simulink model "gpucorr_txsim03r2"  (Simulink 7.4)
settings: Solver=ode3  SolverMode=SingleTasking  StartTime=0.0  StopTime=2^11  RelTol=1e-3
undefined symbols (not defined in the file): sfp
libraries: xbsIndex_r4 x296, xps_library x33, casper_library_misc x2
(part 1 of 2)
settings Model: Creator=gdesvignes  LastModifiedBy=jkocz

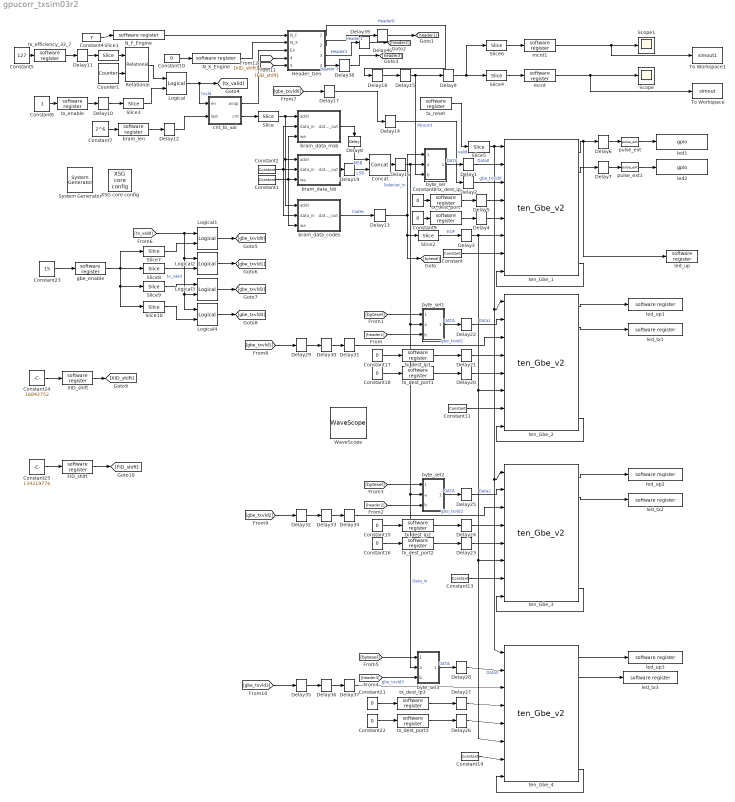
== system gpucorr_txsim03r2 ==
  " System Generator" : xbsIndex_r4/ System Generator  Tag=genX  SystemSampleTime=-1  xilinxfamily=virtex6  part=xc6vsx475t  speed=-1  package=ff1759  synthesis_tool=XST  clock_wrapper=Clock Enables  directory=./gpucorr_txsim03r2/sysgen  testbench=off  simulink_period=1  sysclk_period=5  dcm_input_clock_period=100  incr_netlist=off  trim_vbits=Everywhere in SubSystem  dbl_ovrd=According to Block Masks  core_generation=According to Block Masks  run_coregen=off  deprecated_control=off  eval_field=0  block_type=sysgen
      settings: block_version=11.4
  Concat : xbsIndex_r4/Concat  num_inputs=2  dbl_ovrd=off  block_type=concat
  Constant{,1,11,13,19} (5 alike) : xbsIndex_r4/Constant  arith_type=Boolean  const=0  n_bits=16  bin_pt=14  explicit_period=off  period=1  equ=P=C  opselect=C  inp2=PCIN>>17  opr=+  inp1=P  carry=CIN  dbl_ovrd=off  block_type=constant
      settings: block_version=11.4
  Constant{8..10,15..18,21..22} (9 alike) : Constant  Value=0
  Constant2 : xbsIndex_r4/Constant  arith_type=Unsigned  const=0  n_bits=32  bin_pt=0  explicit_period=off  period=1  equ=P=C  opselect=C  inp2=PCIN>>17  opr=+  inp1=P  carry=CIN  dbl_ovrd=off  block_type=constant
      settings: block_version=11.4
  Constant23 : Constant  Value=15
  Constant24 : Constant  Value=16842752
  Constant25 : Constant  Value=134219776
  Constant4 : Constant  Value=7
  Constant5 : Constant  Value=127
  Constant6 : Constant
  Constant7 : Constant  Value=2^6
  Counter1 : xbsIndex_r4/Counter  cnt_type=Free Running  cnt_to=Inf  operation=Up  start_count=0  cnt_by_val=1  arith_type=Unsigned  n_bits=7  bin_pt=0  load_pin=off  rst=off  en=off  explicit_period=on  period=1  dbl_ovrd=off  use_behavioral_HDL=off  implementation=Fabric  block_type=counter
      settings: block_version=11.4
  Delay{1..3,8,15,19,22,25,28,31,34,37..40} (15 alike) : xbsIndex_r4/Delay  en=off  latency=1  dbl_ovrd=off  reg_retiming=off  block_type=delay
      settings: block_version=11.4
  Delay{4..7,9..12,14,16..18,20..21,23..24,26..27,29..30,32..33,35..36} (24 alike) : xbsIndex_r4/Delay  en=off  latency=2  dbl_ovrd=off  reg_retiming=off  block_type=delay
      settings: block_version=11.4
  Delay13 : xbsIndex_r4/Delay  en=off  latency=3  dbl_ovrd=off  reg_retiming=off  block_type=delay
      settings: block_version=11.4
  FID_shift : xps_library/software register  Tag=xps:sw_reg  SystemSampleTime=-1  io_dir=From Processor  arith_type=Unsigned  bitwidth=32  bin_pt=0  sample_period=1  gw_name=gpucorr_txsim03r2_FID_shift_user_data_out
      link override gpucorr_txsim_tx_enable_user_data_out: arith_type=Unsigned  n_bits=32  bin_pt=0  period=1
  Header_Gen : Subsystem
  Logical{,1..4} (5 alike) : xbsIndex_r4/Logical  logical_function=AND  inputs=2  en=off  latency=0  precision=Full  arith_type=Unsigned  n_bits=16  bin_pt=0  align_bp=on  dbl_ovrd=off  block_type=logical
      settings: block_version=11.4
  N_F_Engine : xps_library/software register  Tag=xps:sw_reg  SystemSampleTime=-1  io_dir=From Processor  arith_type=Unsigned  bitwidth=32  bin_pt=0  sample_period=1  gw_name=gpucorr_txsim03r2_N_F_Engine_user_data_out
      link override gpucorr_txsim_N_F_Engine_user_data_out: arith_type=Unsigned  n_bits=32  bin_pt=0  period=1
  N_X_Engine : xps_library/software register  Tag=xps:sw_reg  SystemSampleTime=-1  io_dir=From Processor  arith_type=Unsigned  bitwidth=32  bin_pt=0  sample_period=1  gw_name=gpucorr_txsim03r2_N_X_Engine_user_data_out
      link override gpucorr_txsim_N_X_Engine_user_data_out: arith_type=Unsigned  n_bits=32  bin_pt=0  period=1
  Relational : xbsIndex_r4/Relational  mode=a>b  en=off  latency=1  dbl_ovrd=off  block_type=relational
  Scope : Scope
  Scope1 : Scope
      settings: TimeRange=100  YMin=-1  YMax=1
  Slice : xbsIndex_r4/Slice  nbits=15  boolean_output=off  mode=Lower Bit Location + Width  bit1=0  base1=MSB of Input  bit0=0  base0=LSB of Input  dbl_ovrd=off  block_type=slice
  Slice1 : xbsIndex_r4/Slice  nbits=7  boolean_output=off  mode=Lower Bit Location + Width  bit1=0  base1=MSB of Input  bit0=0  base0=LSB of Input  dbl_ovrd=off  block_type=slice
  Slice10 : xbsIndex_r4/Slice  nbits=15  boolean_output=on  mode=Lower Bit Location + Width  bit1=0  base1=MSB of Input  bit0=3  base0=LSB of Input  dbl_ovrd=off  block_type=slice
  Slice2 : xbsIndex_r4/Slice  nbits=15  boolean_output=on  mode=Upper Bit Location + Width  bit1=0  base1=MSB of Input  bit0=0  base0=LSB of Input  dbl_ovrd=off  block_type=slice
  Slice3 : xbsIndex_r4/Slice  nbits=15  boolean_output=on  mode=Lower Bit Location + Width  bit1=0  base1=MSB of Input  bit0=0  base0=LSB of Input  dbl_ovrd=off  block_type=slice
  Slice4 : xbsIndex_r4/Slice  nbits=32  boolean_output=off  mode=Lower Bit Location + Width  bit1=0  base1=MSB of Input  bit0=0  base0=LSB of Input  dbl_ovrd=off  block_type=slice
  Slice5 : xbsIndex_r4/Slice  nbits=15  boolean_output=on  mode=Lower Bit Location + Width  bit1=0  base1=MSB of Input  bit0=0  base0=LSB of Input  dbl_ovrd=off  block_type=slice
  Slice6 : xbsIndex_r4/Slice  nbits=32  boolean_output=off  mode=Upper Bit Location + Width  bit1=0  base1=MSB of Input  bit0=0  base0=MSB of Input  dbl_ovrd=off  block_type=slice
  Slice7 : xbsIndex_r4/Slice  nbits=15  boolean_output=on  mode=Lower Bit Location + Width  bit1=0  base1=MSB of Input  bit0=0  base0=LSB of Input  dbl_ovrd=off  block_type=slice
  Slice8 : xbsIndex_r4/Slice  nbits=15  boolean_output=on  mode=Lower Bit Location + Width  bit1=0  base1=MSB of Input  bit0=1  base0=LSB of Input  dbl_ovrd=off  block_type=slice
  Slice9 : xbsIndex_r4/Slice  nbits=15  boolean_output=on  mode=Lower Bit Location + Width  bit1=0  base1=MSB of Input  bit0=2  base0=LSB of Input  dbl_ovrd=off  block_type=slice
  To Workspace : ToWorkspace  VariableName=simout  SampleTime=-1  SaveFormat=Structure
  To Workspace1 : ToWorkspace  VariableName=simout1  SampleTime=-1  SaveFormat=Structure
  WaveScope : xbsIndex_r4/WaveScope  block_type=wavescope
      settings: block_version=11.4
  XID_shift : xps_library/software register  Tag=xps:sw_reg  SystemSampleTime=-1  io_dir=From Processor  arith_type=Unsigned  bitwidth=32  bin_pt=0  sample_period=1  gw_name=gpucorr_txsim03r2_XID_shift_user_data_out
      link override gpucorr_txsim_tx_enable_user_data_out: arith_type=Unsigned  n_bits=32  bin_pt=0  period=1
  XSG core config : xps_library/XSG core config  Tag=xps:xsg  SystemSampleTime=-1  hw_sys=ROACH2:sx475t  clk_src=sys_clk  ROACH_clk_src=sys_clk2x  ROACH2_clk_src=sys_clk  clk_rate=200  sample_period=1  synthesis_tool=XST
  bram_data_codes : Subsystem  Tag=xps:bram  AncestorBlock=xps_library/Shared BRAM  mask{arith_type=Unsigned, addr_width=12, data_width=32, data_bin_pt=0, init_vals=[255,2147483648], sample_rate=1}
      mask prompts: arith_type "Output Data Type"; addr_width "Address width"; data_width "Data Width"; data_bin_pt "Data Binary Point"; init_vals "Initial 32-bit values (simulation only)"; sample_rate "Sample rate"
      mask init:
      | shared_bram_mask;
      mask StyleString: popup(Unsigned|Signed  (2's comp)),edit,popup(8|16|32|64|128),edit,edit,edit
  bram_data_lsb : Subsystem  Tag=xps:bram  AncestorBlock=xps_library/Shared BRAM  mask{arith_type=Unsigned, addr_width=12, data_width=32, data_bin_pt=0, init_vals=[216,212,216], sample_rate=1}
      mask prompts: arith_type "Output Data Type"; addr_width "Address width"; data_width "Data Width"; data_bin_pt "Data Binary Point"; init_vals "Initial 32-bit values (simulation only)"; sample_rate "Sample rate"
      mask init:
      | shared_bram_mask;
      mask StyleString: popup(Unsigned|Signed  (2's comp)),edit,popup(8|16|32|64|128),edit,edit,edit
  bram_data_msb : Subsystem  Tag=xps:bram  AncestorBlock=xps_library/Shared BRAM  mask{arith_type=Unsigned, addr_width=12, data_width=32, data_bin_pt=0, init_vals=[116,112,116], sample_rate=1}
      mask prompts: arith_type "Output Data Type"; addr_width "Address width"; data_width "Data Width"; data_bin_pt "Data Binary Point"; init_vals "Initial 32-bit values (simulation only)"; sample_rate "Sample rate"
      mask init:
      | shared_bram_mask;
      mask StyleString: popup(Unsigned|Signed  (2's comp)),edit,popup(8|16|32|64|128),edit,edit,edit
  bram_len : xps_library/software register  Tag=xps:sw_reg  SystemSampleTime=-1  io_dir=From Processor  arith_type=Unsigned  bitwidth=32  bin_pt=0  sample_period=1  gw_name=gpucorr_txsim03r2_bram_len_user_data_out
      link override gpucorr_txsim_bram_len_user_data_out: arith_type=Unsigned  n_bits=32  bin_pt=0  period=1
  byte_sel : Subsystem
  byte_sel1 : Subsystem
  byte_sel2 : Subsystem
  byte_sel3 : Subsystem
  cnt_to_val : Subsystem
  gbe_enable : xps_library/software register  Tag=xps:sw_reg  SystemSampleTime=-1  io_dir=From Processor  arith_type=Unsigned  bitwidth=32  bin_pt=0  sample_period=1  gw_name=gpucorr_txsim03r2_gbe_enable_user_data_out
      link override gpucorr_txsim_tx_enable_user_data_out: arith_type=Unsigned  n_bits=32  bin_pt=0  period=1
  led1 : xps_library/gpio  Tag=xps:gpio  SystemSampleTime=-1  io_group=ROACH:led  io_dir=out  arith_type=Boolean  bitwidth=1  bin_pt=0  bit_index=1  sample_period=1  use_single_ended=off  use_ddr=off  reg_iob=on  reg_clk_phase=0  termination=None
      link override convert: arith_type=Boolean  n_bits=1  bin_pt=0
  led2 : xps_library/gpio  Tag=xps:gpio  SystemSampleTime=-1  io_group=ROACH:led  io_dir=out  arith_type=Boolean  bitwidth=1  bin_pt=0  bit_index=2  sample_period=1  use_single_ended=off  use_ddr=off  reg_iob=on  reg_clk_phase=0  termination=None
      link override convert: arith_type=Boolean  n_bits=1  bin_pt=0
  led_tx1 : xps_library/software register  Tag=xps:sw_reg  SystemSampleTime=-1  io_dir=To Processor  arith_type=Unsigned  bitwidth=32  bin_pt=0  sample_period=1  gw_name=gpucorr_txsim03r2_led_tx1_user_data_in
      link override convert: arith_type=Unsigned  n_bits=32  bin_pt=0
  led_tx2 : xps_library/software register  Tag=xps:sw_reg  SystemSampleTime=-1  io_dir=To Processor  arith_type=Unsigned  bitwidth=32  bin_pt=0  sample_period=1  gw_name=gpucorr_txsim03r2_led_tx2_user_data_in
      link override convert: arith_type=Unsigned  n_bits=32  bin_pt=0
  led_tx3 : xps_library/software register  Tag=xps:sw_reg  SystemSampleTime=-1  io_dir=To Processor  arith_type=Unsigned  bitwidth=32  bin_pt=0  sample_period=1  gw_name=gpucorr_txsim03r2_led_tx3_user_data_in
      link override convert: arith_type=Unsigned  n_bits=32  bin_pt=0
  led_up : xps_library/software register  Tag=xps:sw_reg  SystemSampleTime=-1  io_dir=To Processor  arith_type=Unsigned  bitwidth=32  bin_pt=0  sample_period=1  gw_name=gpucorr_txsim03r2_led_up_user_data_in
      link override convert: arith_type=Unsigned  n_bits=32  bin_pt=0
  led_up1 : xps_library/software register  Tag=xps:sw_reg  SystemSampleTime=-1  io_dir=To Processor  arith_type=Unsigned  bitwidth=32  bin_pt=0  sample_period=1  gw_name=gpucorr_txsim03r2_led_up1_user_data_in
      link override convert: arith_type=Unsigned  n_bits=32  bin_pt=0
  led_up2 : xps_library/software register  Tag=xps:sw_reg  SystemSampleTime=-1  io_dir=To Processor  arith_type=Unsigned  bitwidth=32  bin_pt=0  sample_period=1  gw_name=gpucorr_txsim03r2_led_up2_user_data_in
      link override convert: arith_type=Unsigned  n_bits=32  bin_pt=0
  led_up3 : xps_library/software register  Tag=xps:sw_reg  SystemSampleTime=-1  io_dir=To Processor  arith_type=Unsigned  bitwidth=32  bin_pt=0  sample_period=1  gw_name=gpucorr_txsim03r2_led_up3_user_data_in
      link override convert: arith_type=Unsigned  n_bits=32  bin_pt=0
  mcnt : xps_library/software register  Tag=xps:sw_reg  SystemSampleTime=-1  io_dir=To Processor  arith_type=Unsigned  bitwidth=32  bin_pt=0  sample_period=1  gw_name=gpucorr_txsim03r2_mcnt_user_data_in
      link override convert: arith_type=Unsigned  n_bits=32  bin_pt=0
  mcnt1 : xps_library/software register  Tag=xps:sw_reg  SystemSampleTime=-1  io_dir=To Processor  arith_type=Unsigned  bitwidth=32  bin_pt=0  sample_period=1  gw_name=gpucorr_txsim03r2_mcnt1_user_data_in
      link override convert: arith_type=Unsigned  n_bits=32  bin_pt=0
  pulse_ext : casper_library_misc/pulse_ext  SystemSampleTime=-1  pulse_len=5
  pulse_ext1 : casper_library_misc/pulse_ext  SystemSampleTime=-1  pulse_len=5
  ten_Gbe_1 : xps_library/ten_Gbe_v2  Tag=xps:tengbe_v2  SystemSampleTime=-1  flavour=sfp+  slot=0  port_r1=0  port_r2_cx4=0  port_r2_sfpp=0  rx_dist_ram=on  large_frames=on  show_param=on  pre_emph_r2=0.74  pre_emph=3  post_emph_r2=0.18  rxeqmix_r2=7  swing_r2=940  swing=800  fab_en=on  fab_mac=hex2dec('123456780000')  fab_ip=192*(2^24) + 168*(2^16) + 5*(2^8) + 20*(2^0)  fab_udp=10000  fab_gate=1  cpu_rx_en=on  cpu_tx_en=on
  ten_Gbe_2 : xps_library/ten_Gbe_v2  Tag=xps:tengbe_v2  SystemSampleTime=-1  flavour=sfp+  slot=0  port_r1=0  port_r2_cx4=0  port_r2_sfpp=1  rx_dist_ram=on  large_frames=on  show_param=on  pre_emph_r2=0.74  pre_emph=3  post_emph_r2=0.18  rxeqmix_r2=7  swing_r2=940  swing=800  fab_en=on  fab_mac=hex2dec('123456789000')  fab_ip=192*(2^24) + 168*(2^16) + 5*(2^8) + 21*(2^0)  fab_udp=10001  fab_gate=1  cpu_rx_en=on  cpu_tx_en=on
  ten_Gbe_3 : xps_library/ten_Gbe_v2  Tag=xps:tengbe_v2  SystemSampleTime=-1  flavour=sfp+  slot=0  port_r1=0  port_r2_cx4=0  port_r2_sfpp=2  rx_dist_ram=on  large_frames=on  show_param=on  pre_emph_r2=0.74  pre_emph=3  post_emph_r2=0.18  rxeqmix_r2=7  swing_r2=940  swing=800  fab_en=on  fab_mac=hex2dec('123456780900')  fab_ip=192*(2^24) + 168*(2^16) + 5*(2^8) + 22*(2^0)  fab_udp=10002  fab_gate=1  cpu_rx_en=on  cpu_tx_en=on
  ten_Gbe_4 : xps_library/ten_Gbe_v2  Tag=xps:tengbe_v2  SystemSampleTime=-1  flavour=sfp+  slot=0  port_r1=0  port_r2_cx4=0  port_r2_sfpp=3  rx_dist_ram=on  large_frames=on  show_param=on  pre_emph_r2=0.74  pre_emph=3  post_emph_r2=0.18  rxeqmix_r2=7  swing_r2=940  swing=800  fab_en=on  fab_mac=hex2dec('123456780090')  fab_ip=192*(2^24) + 168*(2^16) + 5*(2^8) + 23*(2^0)  fab_udp=10003  fab_gate=1  cpu_rx_en=on  cpu_tx_en=on
  tx_dest_ip : xps_library/software register  Tag=xps:sw_reg  SystemSampleTime=-1  io_dir=From Processor  arith_type=Unsigned  bitwidth=32  bin_pt=0  sample_period=1  gw_name=gpucorr_txsim03r2_tx_dest_ip_user_data_out
      link override gpucorr_txsim_tx_dest_ip_user_data_out: arith_type=Unsigned  n_bits=32  bin_pt=0  period=1
  tx_dest_ip1 : xps_library/software register  Tag=xps:sw_reg  SystemSampleTime=-1  io_dir=From Processor  arith_type=Unsigned  bitwidth=32  bin_pt=0  sample_period=1  gw_name=gpucorr_txsim03r2_tx_dest_ip1_user_data_out
      link override gpucorr_txsim_tx_dest_ip_user_data_out: arith_type=Unsigned  n_bits=32  bin_pt=0  period=1
  tx_dest_ip2 : xps_library/software register  Tag=xps:sw_reg  SystemSampleTime=-1  io_dir=From Processor  arith_type=Unsigned  bitwidth=32  bin_pt=0  sample_period=1  gw_name=gpucorr_txsim03r2_tx_dest_ip2_user_data_out
      link override gpucorr_txsim_tx_dest_ip_user_data_out: arith_type=Unsigned  n_bits=32  bin_pt=0  period=1
  tx_dest_ip3 : xps_library/software register  Tag=xps:sw_reg  SystemSampleTime=-1  io_dir=From Processor  arith_type=Unsigned  bitwidth=32  bin_pt=0  sample_period=1  gw_name=gpucorr_txsim03r2_tx_dest_ip3_user_data_out
      link override gpucorr_txsim_tx_dest_ip_user_data_out: arith_type=Unsigned  n_bits=32  bin_pt=0  period=1
  tx_dest_port : xps_library/software register  Tag=xps:sw_reg  SystemSampleTime=-1  io_dir=From Processor  arith_type=Unsigned  bitwidth=32  bin_pt=0  sample_period=1  gw_name=gpucorr_txsim03r2_tx_dest_port_user_data_out
      link override gpucorr_txsim_tx_dest_port_user_data_out: arith_type=Unsigned  n_bits=32  bin_pt=0  period=1
  tx_dest_port1 : xps_library/software register  Tag=xps:sw_reg  SystemSampleTime=-1  io_dir=From Processor  arith_type=Unsigned  bitwidth=32  bin_pt=0  sample_period=1  gw_name=gpucorr_txsim03r2_tx_dest_port1_user_data_out
      link override gpucorr_txsim_tx_dest_port_user_data_out: arith_type=Unsigned  n_bits=32  bin_pt=0  period=1
  tx_dest_port2 : xps_library/software register  Tag=xps:sw_reg  SystemSampleTime=-1  io_dir=From Processor  arith_type=Unsigned  bitwidth=32  bin_pt=0  sample_period=1  gw_name=gpucorr_txsim03r2_tx_dest_port2_user_data_out
      link override gpucorr_txsim_tx_dest_port_user_data_out: arith_type=Unsigned  n_bits=32  bin_pt=0  period=1
  tx_dest_port3 : xps_library/software register  Tag=xps:sw_reg  SystemSampleTime=-1  io_dir=From Processor  arith_type=Unsigned  bitwidth=32  bin_pt=0  sample_period=1  gw_name=gpucorr_txsim03r2_tx_dest_port3_user_data_out
      link override gpucorr_txsim_tx_dest_port_user_data_out: arith_type=Unsigned  n_bits=32  bin_pt=0  period=1
  tx_efficiency_32_7 : xps_library/software register  Tag=xps:sw_reg  SystemSampleTime=-1  io_dir=From Processor  arith_type=Unsigned  bitwidth=32  bin_pt=0  sample_period=1  gw_name=gpucorr_txsim03r2_tx_efficiency_32_7_user_data_out
      link override gpucorr_txsim_tx_efficiency_32_7_user_data_out: arith_type=Unsigned  n_bits=32  bin_pt=0  period=1
  tx_enable : xps_library/software register  Tag=xps:sw_reg  SystemSampleTime=-1  io_dir=From Processor  arith_type=Unsigned  bitwidth=32  bin_pt=0  sample_period=1  gw_name=gpucorr_txsim03r2_tx_enable_user_data_out
      link override gpucorr_txsim_tx_enable_user_data_out: arith_type=Unsigned  n_bits=32  bin_pt=0  period=1
  tx_reset : xps_library/software register  Tag=xps:sw_reg  SystemSampleTime=-1  io_dir=From Processor  arith_type=Unsigned  bitwidth=32  bin_pt=0  sample_period=1  gw_name=gpucorr_txsim03r2_tx_reset_user_data_out
      link override gpucorr_txsim_tx_reset_user_data_out: arith_type=Unsigned  n_bits=32  bin_pt=0  period=1
  wires:
  tx_dest_ip/1 -> Delay5/1
  tx_dest_port/1 -> Delay4/1
  Slice/1 -> bram_data_lsb/1(addr), bram_data_codes/1(addr), bram_data_msb/1(addr)
  Constant1/1 -> bram_data_lsb/3(we), bram_data_msb/3(we), bram_data_codes/3(we)
  Constant2/1 -> bram_data_lsb/2(data_in), bram_data_msb/2(data_in), bram_data_codes/2(data_in)
  bram_data_msb/1(data_out) -> Delay8/1
  tx_efficiency_32_7/1 -> Delay11/1
  Slice1/1 -> Relational/1
  Counter1/1 -> Relational/2
  bram_len/1 -> Delay12/1
  cnt_to_val/1(wrap) -> Header_Gen/3(En)
  Concat/1 -> Delay16/1
  bram_data_codes/1(data_out) -> Delay13/1  "Codes"
  byte_sel/1(dout) -> Delay1/1  "DATA"
  Delay17/1 -> Delay14/1
  Slice2/1 -> Delay3/1  "EOF"
  tx_enable/1 -> Delay10/1
  Logical/1 -> cnt_to_val/1(en), [tx_valid]  "txvld"
  Relational/1 -> Logical/1
  Slice3/1 -> Logical/2
  Constant5/1 -> tx_efficiency_32_7/1
  Constant6/1 -> tx_enable/1
  Constant7/1 -> bram_len/1
  Constant8/1 -> tx_dest_ip/1
  Constant9/1 -> tx_dest_port/1
  Slice4/1 -> mcnt/1
  Delay6/1 -> pulse_ext/1
  Delay7/1 -> pulse_ext1/1
  Delay9/1 -> Slice4/1, Slice6/1
  Delay10/1 -> Slice3/1
  Delay11/1 -> Slice1/1
  Delay12/1 -> cnt_to_val/2(last)
  Delay13/1 -> byte_sel/1(byte_sel), Slice2/1, [bytesel]  "Selecter_in"
  Delay14/1 -> Delay2/1  "valid"
  Delay15/1 -> byte_sel/3(b), Delay9/1  "Mcount"
  Delay16/1 -> byte_sel1/2(a), byte_sel2/2(a), byte_sel3/2(a), byte_sel/2(a)  "Data_in"
  Delay18/1 -> Delay15/1
  tx_reset/1 -> Slice5/1
  Slice5/1 -> ten_Gbe_4/1, ten_Gbe_3/1, ten_Gbe_2/1, ten_Gbe_1/1
  Constant/1 -> ten_Gbe_1/7
  Delay1/1 -> ten_Gbe_1/2  "Data0"
  Delay2/1 -> ten_Gbe_1/3  "gbe_txvld0"
  ten_Gbe_1/1 -> Delay6/1, led_up/1
  pulse_ext/1 -> led1/1
  pulse_ext1/1 -> led2/1
  Delay5/1 -> ten_Gbe_1/4
  Delay4/1 -> ten_Gbe_1/5
  Delay3/1 -> ten_Gbe_4/6, ten_Gbe_3/6, ten_Gbe_2/6, ten_Gbe_1/6
  ten_Gbe_1/3 -> Delay7/1
  cnt_to_val/2(cnt) -> Slice/1
  Constant4/1 -> N_F_Engine/1
  Constant10/1 -> N_X_Engine/1
  N_X_Engine/1 -> Header_Gen/2(N_X)
  Header_Gen/1(Header) -> Delay18/1  "Header0"
  mcnt/1 -> Scope/1, To Workspace/1
  Slice6/1 -> mcnt1/1
  mcnt1/1 -> Scope1/1, To Workspace1/1
  Delay8/1 -> Concat/1  "MSB"
  bram_data_lsb/1(data_out) -> Delay19/1
  Delay19/1 -> Concat/2  "LSB"
  Constant11/1 -> ten_Gbe_2/7
  tx_dest_ip1/1 -> Delay21/1
  tx_dest_port1/1 -> Delay20/1
  Constant17/1 -> tx_dest_ip1/1
  Constant18/1 -> tx_dest_port1/1
  Delay21/1 -> ten_Gbe_2/4
  Delay20/1 -> ten_Gbe_2/5
  ten_Gbe_2/1 -> led_up1/1
  ten_Gbe_2/3 -> led_tx1/1
  byte_sel1/1(dout) -> Delay22/1  "DATA"
  Delay22/1 -> ten_Gbe_2/2  "Data1"
  [bytesel] -> byte_sel1/1(byte_sel)
  [header1] -> byte_sel1/3(b)
  N_F_Engine/1 -> Header_Gen/1(N_F)
  Constant13/1 -> ten_Gbe_3/7
  tx_dest_ip2/1 -> Delay24/1
  tx_dest_port2/1 -> Delay23/1
  Constant15/1 -> tx_dest_ip2/1
  Constant16/1 -> tx_dest_port2/1
  Delay24/1 -> ten_Gbe_3/4
  Delay23/1 -> ten_Gbe_3/5
  ten_Gbe_3/1 -> led_up2/1
  ten_Gbe_3/3 -> led_tx2/1
  byte_sel2/1(dout) -> Delay25/1  "DATA"
  Delay25/1 -> ten_Gbe_3/2  "Data2"
  [bytesel] -> byte_sel2/1(byte_sel)
  [header2] -> byte_sel2/3(b)
  Constant19/1 -> ten_Gbe_4/7
  tx_dest_ip3/1 -> Delay27/1
  tx_dest_port3/1 -> Delay26/1
  Constant21/1 -> tx_dest_ip3/1
  Constant22/1 -> tx_dest_port3/1
  Delay27/1 -> ten_Gbe_4/4
  Delay26/1 -> ten_Gbe_4/5
  ten_Gbe_4/1 -> led_up3/1
  byte_sel3/1(dout) -> Delay28/1  "DATA"
  Delay28/1 -> ten_Gbe_4/2  "Data3"
  [bytesel] -> byte_sel3/1(byte_sel)
  [header3] -> byte_sel3/3(b)
  Constant23/1 -> gbe_enable/1
  gbe_enable/1 -> Slice7/1, Slice8/1, Slice9/1, Slice10/1
  Slice7/1 -> Logical1/2
  Slice8/1 -> Logical2/2
  Slice9/1 -> Logical3/1
  Slice10/1 -> Logical4/2
  [tx_valid] -> Logical1/1, Logical2/1, Logical3/2, Logical4/1  "tx_valid"
  Logical1/1 -> [gbe_txvld0]
  Logical2/1 -> [gbe_txvld1]
  Logical3/1 -> [gbe_txvld2]
  Logical4/1 -> [gbe_txvld3]
  [gbe_txvld0] -> Delay17/1
  [gbe_txvld1] -> Delay29/1
  Delay29/1 -> Delay30/1
  Delay30/1 -> Delay31/1
  [gbe_txvld2] -> Delay32/1
  Delay32/1 -> Delay33/1
  Delay33/1 -> Delay34/1
  [gbe_txvld3] -> Delay35/1
  Delay35/1 -> Delay36/1
  Delay36/1 -> Delay37/1
  Delay31/1 -> ten_Gbe_2/3  "gbe_txvld1"
  Delay34/1 -> ten_Gbe_3/3  "gbe_txvld2"
  Delay37/1 -> ten_Gbe_4/3  "gbe_txvld3"
  Delay38/1 -> [header3]
  Header_Gen/4(Header3) -> Delay38/1  "Header 3"
  Delay40/1 -> [header1]
  Header_Gen/2(Header1) -> Delay40/1  "Header1"
  Header_Gen/3(Header2) -> Delay39/1  "Header2"
  Delay39/1 -> [header2]
  [FID_shift] -> Header_Gen/4(FID_shift)
  [XID_shift] -> Header_Gen/5(XID_shift)
  XID_shift/1 -> [XID_shift]
  FID_shift/1 -> [FID_shift]
  Constant24/1 -> XID_shift/1
  Constant25/1 -> FID_shift/1
  ten_Gbe_4/3 -> led_tx3/1
  ten_Gbe_4/12 -> ten_Gbe_4/8
  ten_Gbe_3/12 -> ten_Gbe_3/8
  ten_Gbe_2/12 -> ten_Gbe_2/8
  ten_Gbe_1/12 -> ten_Gbe_1/8

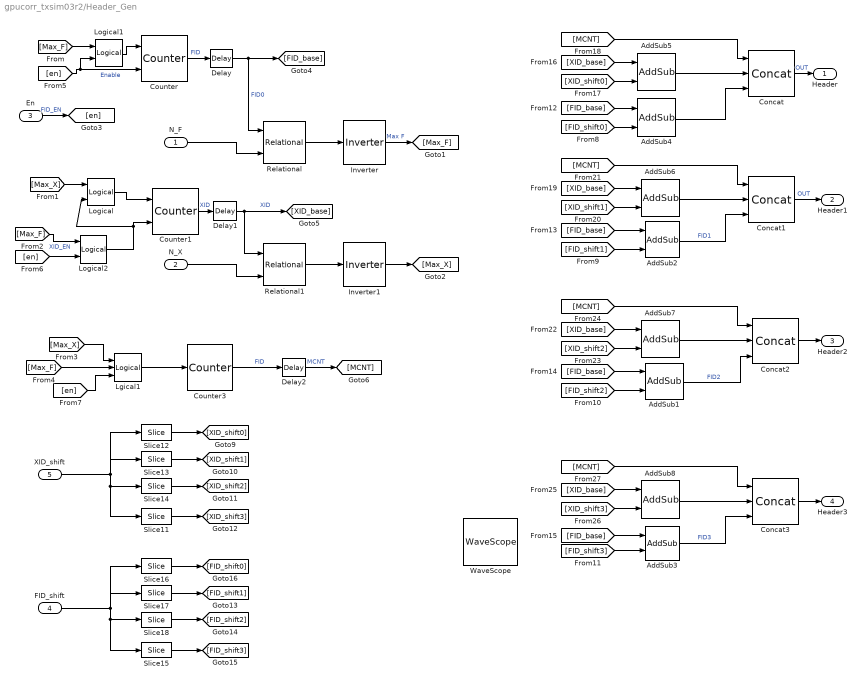
== system gpucorr_txsim03r2/Header_Gen ==
  N_F : Inport
  N_X : Inport  Port=2
  En : Inport  Port=3
  FID_shift : Inport  Port=4
  XID_shift : Inport  Port=5
  AddSub{1..8} (8 alike) : xbsIndex_r4/AddSub  mode=Addition  use_carryin=off  use_carryout=off  en=off  latency=0  precision=User Defined  arith_type=Unsigned  n_bits=8  bin_pt=0  quantization=Truncate  overflow=Wrap  dbl_ovrd=off  use_behavioral_HDL=off  hw_selection=Fabric  pipelined=off  block_type=addsub
  Concat{,1..3} (4 alike) : xbsIndex_r4/Concat  num_inputs=3  dbl_ovrd=off  block_type=concat
  Counter : xbsIndex_r4/Counter  cnt_type=Free Running  cnt_to=Inf  operation=Up  start_count=0  cnt_by_val=1  arith_type=Unsigned  n_bits=8  bin_pt=0  load_pin=off  rst=on  en=on  explicit_period=on  period=1  dbl_ovrd=off  use_behavioral_HDL=off  implementation=Fabric  block_type=counter
      settings: block_version=11.4
  Counter1 : xbsIndex_r4/Counter  cnt_type=Free Running  cnt_to=Inf  operation=Up  start_count=0  cnt_by_val=1  arith_type=Unsigned  n_bits=8  bin_pt=0  load_pin=off  rst=on  en=on  explicit_period=on  period=1  dbl_ovrd=off  use_behavioral_HDL=off  implementation=Fabric  block_type=counter
      settings: block_version=11.4
  Counter3 : xbsIndex_r4/Counter  cnt_type=Free Running  cnt_to=Inf  operation=Up  start_count=0  cnt_by_val=1  arith_type=Unsigned  n_bits=48  bin_pt=0  load_pin=off  rst=off  en=on  explicit_period=on  period=1  dbl_ovrd=off  use_behavioral_HDL=off  implementation=Fabric  block_type=counter
      settings: block_version=11.4
  Delay : xbsIndex_r4/Delay  en=off  latency=1  dbl_ovrd=off  reg_retiming=off  block_type=delay
      settings: block_version=11.4
  Delay1 : xbsIndex_r4/Delay  en=off  latency=1  dbl_ovrd=off  reg_retiming=off  block_type=delay
      settings: block_version=11.4
  Delay2 : xbsIndex_r4/Delay  en=off  latency=1  dbl_ovrd=off  reg_retiming=off  block_type=delay
      settings: block_version=11.4
  Inverter : xbsIndex_r4/Inverter  en=off  latency=0  dbl_ovrd=off  block_type=inv
      settings: block_version=11.4
  Inverter1 : xbsIndex_r4/Inverter  en=off  latency=0  dbl_ovrd=off  block_type=inv
      settings: block_version=11.4
  Lgical1 : xbsIndex_r4/Logical  logical_function=AND  inputs=3  en=off  latency=0  precision=Full  arith_type=Unsigned  n_bits=16  bin_pt=0  align_bp=on  dbl_ovrd=off  block_type=logical
      settings: block_version=11.4
  Logical : xbsIndex_r4/Logical  logical_function=AND  inputs=2  en=off  latency=0  precision=Full  arith_type=Unsigned  n_bits=16  bin_pt=0  align_bp=on  dbl_ovrd=off  block_type=logical
      settings: block_version=11.4
  Logical1 : xbsIndex_r4/Logical  logical_function=AND  inputs=2  en=off  latency=0  precision=Full  arith_type=Unsigned  n_bits=16  bin_pt=0  align_bp=on  dbl_ovrd=off  block_type=logical
      settings: block_version=11.4
  Logical2 : xbsIndex_r4/Logical  logical_function=AND  inputs=2  en=off  latency=0  precision=Full  arith_type=Unsigned  n_bits=16  bin_pt=0  align_bp=on  dbl_ovrd=off  block_type=logical
      settings: block_version=11.4
  Relational : xbsIndex_r4/Relational  mode=a<b  en=off  latency=0  dbl_ovrd=off  block_type=relational
  Relational1 : xbsIndex_r4/Relational  mode=a<b  en=off  latency=0  dbl_ovrd=off  block_type=relational
  Slice11 : xbsIndex_r4/Slice  nbits=8  boolean_output=off  mode=Lower Bit Location + Width  bit1=0  base1=MSB of Input  bit0=24  base0=LSB of Input  dbl_ovrd=off  block_type=slice
  Slice12 : xbsIndex_r4/Slice  nbits=8  boolean_output=off  mode=Lower Bit Location + Width  bit1=0  base1=MSB of Input  bit0=0  base0=LSB of Input  dbl_ovrd=off  block_type=slice
  Slice13 : xbsIndex_r4/Slice  nbits=8  boolean_output=off  mode=Lower Bit Location + Width  bit1=0  base1=MSB of Input  bit0=8  base0=LSB of Input  dbl_ovrd=off  block_type=slice
  Slice14 : xbsIndex_r4/Slice  nbits=8  boolean_output=off  mode=Lower Bit Location + Width  bit1=0  base1=MSB of Input  bit0=16  base0=LSB of Input  dbl_ovrd=off  block_type=slice
  Slice15 : xbsIndex_r4/Slice  nbits=8  boolean_output=off  mode=Lower Bit Location + Width  bit1=0  base1=MSB of Input  bit0=24  base0=LSB of Input  dbl_ovrd=off  block_type=slice
  Slice16 : xbsIndex_r4/Slice  nbits=8  boolean_output=off  mode=Lower Bit Location + Width  bit1=0  base1=MSB of Input  bit0=0  base0=LSB of Input  dbl_ovrd=off  block_type=slice
  Slice17 : xbsIndex_r4/Slice  nbits=8  boolean_output=off  mode=Lower Bit Location + Width  bit1=0  base1=MSB of Input  bit0=8  base0=LSB of Input  dbl_ovrd=off  block_type=slice
  Slice18 : xbsIndex_r4/Slice  nbits=8  boolean_output=off  mode=Lower Bit Location + Width  bit1=0  base1=MSB of Input  bit0=16  base0=LSB of Input  dbl_ovrd=off  block_type=slice
  WaveScope : xbsIndex_r4/WaveScope  block_type=wavescope
      settings: block_version=11.4
  Header : Outport
  Header1 : Outport  Port=2
  Header2 : Outport  Port=3
  Header3 : Outport  Port=4
  wires:
  Counter/1 -> Delay/1  "FID"
  Relational/1 -> Inverter/1
  Counter1/1 -> Delay1/1  "XID"
  Relational1/1 -> Inverter1/1
  N_F/1 -> Relational/2
  Inverter/1 -> [Max_F]  "Max F"
  Inverter1/1 -> [Max_X]
  [Max_F] -> Logical2/1  "XID_EN"
  [Max_X] -> Logical/1
  Logical/1 -> Counter1/1
  [Max_X] -> Lgical1/1
  Concat/1 -> Header/1  "OUT"
  N_X/1 -> Relational1/2
  Counter3/1 -> Delay2/1  "FID"
  En/1 -> [en]  "FID_EN"
  [Max_F] -> Logical1/1
  [en] -> Logical1/2, Counter/2  "Enable"
  Logical1/1 -> Counter/1
  [en] -> Logical2/2
  Logical2/1 -> Counter1/2, Logical/2
  [Max_F] -> Lgical1/2
  [en] -> Lgical1/3
  Delay/1 -> Relational/1, [FID_base]  "FID0"
  Delay1/1 -> Relational1/1, [XID_base]  "XID"
  Lgical1/1 -> Counter3/1
  AddSub2/1 -> Concat1/3  "FID1"
  Concat1/1 -> Header1/1  "OUT"
  AddSub1/1 -> Concat2/3  "FID2"
  AddSub3/1 -> Concat3/3  "FID3"
  Concat2/1 -> Header2/1
  Concat3/1 -> Header3/1
  XID_shift/1 -> Slice12/1, Slice13/1, Slice14/1, Slice11/1
  Slice12/1 -> [XID_shift0]
  Slice13/1 -> [XID_shift1]
  Slice14/1 -> [XID_shift2]
  Slice11/1 -> [XID_shift3]
  FID_shift/1 -> Slice15/1, Slice18/1, Slice17/1, Slice16/1
  Slice16/1 -> [FID_shift0]
  Slice17/1 -> [FID_shift1]
  Slice18/1 -> [FID_shift2]
  Slice15/1 -> [FID_shift3]
  [FID_shift0] -> AddSub4/2
  AddSub4/1 -> Concat/3
  [FID_shift1] -> AddSub2/2
  [FID_shift2] -> AddSub1/2
  [FID_shift3] -> AddSub3/2
  [FID_base] -> AddSub4/1
  [FID_base] -> AddSub2/1
  [FID_base] -> AddSub1/1
  [FID_base] -> AddSub3/1
  Delay2/1 -> [MCNT]  "MCNT"
  [XID_shift0] -> AddSub5/2
  [XID_base] -> AddSub5/1
  AddSub5/1 -> Concat/2
  [MCNT] -> Concat/1
  [XID_shift1] -> AddSub6/2
  [XID_base] -> AddSub6/1
  [MCNT] -> Concat1/1
  AddSub6/1 -> Concat1/2
  [XID_shift2] -> AddSub7/2
  [XID_base] -> AddSub7/1
  [MCNT] -> Concat2/1
  AddSub7/1 -> Concat2/2
  [XID_shift3] -> AddSub8/2
  [XID_base] -> AddSub8/1
  [MCNT] -> Concat3/1
  AddSub8/1 -> Concat3/2

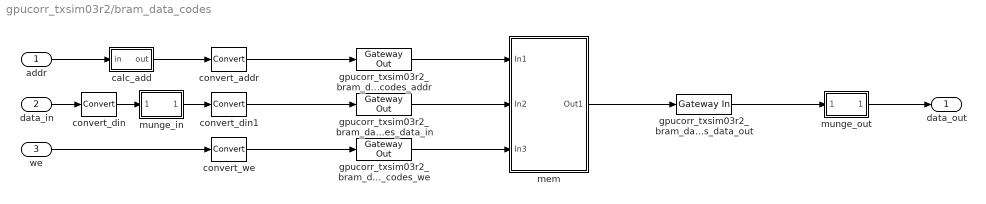
== system gpucorr_txsim03r2/bram_data_codes ==
  addr : Inport
  data_in : Inport  Port=2
  we : Inport  Port=3
  calc_add : Subsystem
  convert_addr : xbsIndex_r4/Convert  arith_type=Unsigned  n_bits=addr_width  bin_pt=0  quantization=Truncate  overflow=Wrap  latency=0  dbl_ovrd=off  pipeline=off  block_type=convert
      settings: xl_area=[0, 0, 0, 0, 0, 0, 0]
  convert_din : xbsIndex_r4/Convert  arith_type=Unsigned  n_bits=data_width  bin_pt=data_bin_pt  quantization=Truncate  overflow=Wrap  latency=0  dbl_ovrd=off  pipeline=off  block_type=convert
      settings: xl_area=[0, 0, 0, 0, 0, 0, 0]
  convert_din1 : xbsIndex_r4/Convert  arith_type=Unsigned  n_bits=data_width  bin_pt=data_bin_pt  quantization=Truncate  overflow=Wrap  latency=0  dbl_ovrd=off  pipeline=off  block_type=convert
      settings: xl_area=[0, 0, 0, 0, 0, 0, 0]
  convert_we : xbsIndex_r4/Convert  arith_type=Unsigned  n_bits=1  bin_pt=0  quantization=Truncate  overflow=Wrap  latency=0  dbl_ovrd=off  pipeline=off  block_type=convert
      settings: xl_area=[0, 0, 0, 0, 0, 0, 0]
  gpucorr_txsim03r2_bram_data_codes_addr : xbsIndex_r4/Gateway Out  hdl_port=on  timing_constraint=None  locs_specified=off  LOCs={'A5','B9','A9','C1','A3','G6','E9','A6','A7','A8','B8','B1','B3','D9','B5','B4','B6','C2'}  block_type=gatewayout
      settings: infoedit="Gateway out block.  Converts Xilinx fixed point inputs into ouputs of type Simulink integer, double, or fixed point.<P><P>Hardware notes:  In hardware these blocks become top level output ports or are discarded, depending on how they are configured."  xl_area=[0, 0, 0, 0, 0, 0, 0]  sginterface={'Nallatech'=>{'xdspkit'=>{'non_memory_mapped_port'=>'uprev_Shared_BRAM_addr'}},'Xilinx'=>{'jtaghwcosim'=>{'non_memory_mapped_port'=>'uprev_Shared_BRAM_addr'},'xdspkit'=>{'non_memory_mapped_port'=>'uprev_Shared_BRAM_addr'}}}
  gpucorr_txsim03r2_bram_data_codes_data_in : xbsIndex_r4/Gateway Out  hdl_port=on  timing_constraint=None  locs_specified=off  LOCs={'B21','B22','A22','B23','B19','C19','A20','A21','A23','B24','A24','A25','E18','D18','C18','B18'}  block_type=gatewayout
      settings: infoedit="Gateway out block.  Converts Xilinx fixed point inputs into ouputs of type Simulink integer, double, or fixed point.<P><P>Hardware notes:  In hardware these blocks become top level output ports or are discarded, depending on how they are configured."  xl_area=[0, 0, 0, 0, 0, 0, 0]  sginterface={'Nallatech'=>{'xdspkit'=>{'non_memory_mapped_port'=>'uprev_Shared_BRAM_data_in'}},'Xilinx'=>{'jtaghwcosim'=>{'non_memory_mapped_port'=>'uprev_Shared_BRAM_data_in'},'xdspkit'=>{'non_memory_mapped_port'=>'uprev_Shared_BRAM_data_in'}}}
  gpucorr_txsim03r2_bram_data_codes_data_out : xbsIndex_r4/Gateway In  arith_type=Unsigned  n_bits=data_width  bin_pt=data_bin_pt  quantization=Truncate  overflow=Wrap  period=sample_rate  dbl_ovrd=off  timing_constraint=None  locs_specified=off  LOCs={}  hdl_port=on  block_type=gatewayin
      settings: infoedit="Gateway in block.  Converts inputs of type Simulink integer, double and fixed point to  Xilinx fixed point type.<br><br>Hardware notes:  In hardware these blocks become top level input ports."  xl_area=[0, 0, 0, 0, 0, 0, 0]
  gpucorr_txsim03r2_bram_data_codes_we : xbsIndex_r4/Gateway Out  hdl_port=on  timing_constraint=None  locs_specified=off  LOCs={'A14'}  block_type=gatewayout
      settings: infoedit="Gateway out block.  Converts Xilinx fixed point inputs into ouputs of type Simulink integer, double, or fixed point.<P><P>Hardware notes:  In hardware these blocks become top level output ports or are discarded, depending on how they are configured."  xl_area=[0, 0, 0, 0, 0, 0, 0]
  mem : Subsystem
  munge_in : Subsystem  AncestorBlock=casper_library_flow_control/munge  mask(munge){divisions=1, div_size=32, order=[0]}
      mask prompts: divisions "Number of divisions"; div_size "Division size (bits)"; order "Division packing order"
      mask help: Splits an input bus into the specified number of divisions and then recombines them in the order specified (most significant division = 0,least = number divisions-1)
      mask init:
      | munge_init(gcb, ...
      |     'divisions', divisions, ...
      |     'div_size', div_size, ...
      |     'order', order);
      settings: AttributesFormatString=|
      | [0]
      | 32 bits
  munge_out : Subsystem  AncestorBlock=casper_library_flow_control/munge  mask(munge){divisions=1, div_size=32, order=[0]}
      mask prompts: divisions "Number of divisions"; div_size "Division size (bits)"; order "Division packing order"
      mask help: Splits an input bus into the specified number of divisions and then recombines them in the order specified (most significant division = 0,least = number divisions-1)
      mask init:
      | munge_init(gcb, ...
      |     'divisions', divisions, ...
      |     'div_size', div_size, ...
      |     'order', order);
      settings: AttributesFormatString=|
      | [0]
      | 32 bits
  data_out : Outport
  wires:
  convert_din/1 -> munge_in/1(din)
  convert_din1/1 -> gpucorr_txsim03r2_bram_data_codes_data_in/1
  convert_addr/1 -> gpucorr_txsim03r2_bram_data_codes_addr/1
  calc_add/1(out) -> convert_addr/1
  munge_out/1(dout) -> data_out/1
  munge_in/1(dout) -> convert_din1/1
  gpucorr_txsim03r2_bram_data_codes_we/1 -> mem/3(In3)
  gpucorr_txsim03r2_bram_data_codes_data_in/1 -> mem/2(In2)
  gpucorr_txsim03r2_bram_data_codes_addr/1 -> mem/1(In1)
  convert_we/1 -> gpucorr_txsim03r2_bram_data_codes_we/1
  we/1 -> convert_we/1
  addr/1 -> calc_add/1(in)
  gpucorr_txsim03r2_bram_data_codes_data_out/1 -> munge_out/1(din)
  data_in/1 -> convert_din/1
  mem/1(Out1) -> gpucorr_txsim03r2_bram_data_codes_data_out/1

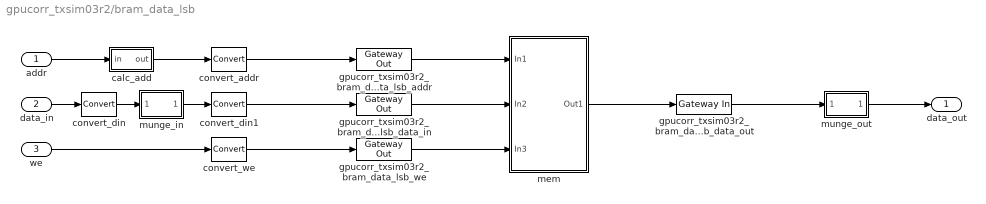
== system gpucorr_txsim03r2/bram_data_lsb ==
  addr : Inport
  data_in : Inport  Port=2
  we : Inport  Port=3
  calc_add : Subsystem
  convert_addr : xbsIndex_r4/Convert  arith_type=Unsigned  n_bits=addr_width  bin_pt=0  quantization=Truncate  overflow=Wrap  latency=0  dbl_ovrd=off  pipeline=off  block_type=convert
      settings: xl_area=[0, 0, 0, 0, 0, 0, 0]
  convert_din : xbsIndex_r4/Convert  arith_type=Unsigned  n_bits=data_width  bin_pt=data_bin_pt  quantization=Truncate  overflow=Wrap  latency=0  dbl_ovrd=off  pipeline=off  block_type=convert
      settings: xl_area=[0, 0, 0, 0, 0, 0, 0]
  convert_din1 : xbsIndex_r4/Convert  arith_type=Unsigned  n_bits=data_width  bin_pt=data_bin_pt  quantization=Truncate  overflow=Wrap  latency=0  dbl_ovrd=off  pipeline=off  block_type=convert
      settings: xl_area=[0, 0, 0, 0, 0, 0, 0]
  convert_we : xbsIndex_r4/Convert  arith_type=Unsigned  n_bits=1  bin_pt=0  quantization=Truncate  overflow=Wrap  latency=0  dbl_ovrd=off  pipeline=off  block_type=convert
      settings: xl_area=[0, 0, 0, 0, 0, 0, 0]
  gpucorr_txsim03r2_bram_data_lsb_addr : xbsIndex_r4/Gateway Out  hdl_port=on  timing_constraint=None  locs_specified=off  LOCs={'A5','B9','A9','C1','A3','G6','E9','A6','A7','A8','B8','B1','B3','D9','B5','B4','B6','C2'}  block_type=gatewayout
      settings: infoedit="Gateway out block.  Converts Xilinx fixed point inputs into ouputs of type Simulink integer, double, or fixed point.<P><P>Hardware notes:  In hardware these blocks become top level output ports or are discarded, depending on how they are configured."  xl_area=[0, 0, 0, 0, 0, 0, 0]  sginterface={'Nallatech'=>{'xdspkit'=>{'non_memory_mapped_port'=>'uprev_Shared_BRAM_addr'}},'Xilinx'=>{'jtaghwcosim'=>{'non_memory_mapped_port'=>'uprev_Shared_BRAM_addr'},'xdspkit'=>{'non_memory_mapped_port'=>'uprev_Shared_BRAM_addr'}}}
  gpucorr_txsim03r2_bram_data_lsb_data_in : xbsIndex_r4/Gateway Out  hdl_port=on  timing_constraint=None  locs_specified=off  LOCs={'B21','B22','A22','B23','B19','C19','A20','A21','A23','B24','A24','A25','E18','D18','C18','B18'}  block_type=gatewayout
      settings: infoedit="Gateway out block.  Converts Xilinx fixed point inputs into ouputs of type Simulink integer, double, or fixed point.<P><P>Hardware notes:  In hardware these blocks become top level output ports or are discarded, depending on how they are configured."  xl_area=[0, 0, 0, 0, 0, 0, 0]  sginterface={'Nallatech'=>{'xdspkit'=>{'non_memory_mapped_port'=>'uprev_Shared_BRAM_data_in'}},'Xilinx'=>{'jtaghwcosim'=>{'non_memory_mapped_port'=>'uprev_Shared_BRAM_data_in'},'xdspkit'=>{'non_memory_mapped_port'=>'uprev_Shared_BRAM_data_in'}}}
  gpucorr_txsim03r2_bram_data_lsb_data_out : xbsIndex_r4/Gateway In  arith_type=Unsigned  n_bits=data_width  bin_pt=data_bin_pt  quantization=Truncate  overflow=Wrap  period=sample_rate  dbl_ovrd=off  timing_constraint=None  locs_specified=off  LOCs={}  hdl_port=on  block_type=gatewayin
      settings: infoedit="Gateway in block.  Converts inputs of type Simulink integer, double and fixed point to  Xilinx fixed point type.<br><br>Hardware notes:  In hardware these blocks become top level input ports."  xl_area=[0, 0, 0, 0, 0, 0, 0]
  gpucorr_txsim03r2_bram_data_lsb_we : xbsIndex_r4/Gateway Out  hdl_port=on  timing_constraint=None  locs_specified=off  LOCs={'A14'}  block_type=gatewayout
      settings: infoedit="Gateway out block.  Converts Xilinx fixed point inputs into ouputs of type Simulink integer, double, or fixed point.<P><P>Hardware notes:  In hardware these blocks become top level output ports or are discarded, depending on how they are configured."  xl_area=[0, 0, 0, 0, 0, 0, 0]
  mem : Subsystem
  munge_in : Subsystem  AncestorBlock=casper_library_flow_control/munge  mask(munge){divisions=1, div_size=32, order=[0]}
      mask prompts: divisions "Number of divisions"; div_size "Division size (bits)"; order "Division packing order"
      mask help: Splits an input bus into the specified number of divisions and then recombines them in the order specified (most significant division = 0,least = number divisions-1)
      mask init:
      | munge_init(gcb, ...
      |     'divisions', divisions, ...
      |     'div_size', div_size, ...
      |     'order', order);
      settings: AttributesFormatString=|
      | [0]
      | 32 bits
  munge_out : Subsystem  AncestorBlock=casper_library_flow_control/munge  mask(munge){divisions=1, div_size=32, order=[0]}
      mask prompts: divisions "Number of divisions"; div_size "Division size (bits)"; order "Division packing order"
      mask help: Splits an input bus into the specified number of divisions and then recombines them in the order specified (most significant division = 0,least = number divisions-1)
      mask init:
      | munge_init(gcb, ...
      |     'divisions', divisions, ...
      |     'div_size', div_size, ...
      |     'order', order);
      settings: AttributesFormatString=|
      | [0]
      | 32 bits
  data_out : Outport
  wires:
  convert_din/1 -> munge_in/1(din)
  convert_din1/1 -> gpucorr_txsim03r2_bram_data_lsb_data_in/1
  convert_addr/1 -> gpucorr_txsim03r2_bram_data_lsb_addr/1
  calc_add/1(out) -> convert_addr/1
  munge_out/1(dout) -> data_out/1
  munge_in/1(dout) -> convert_din1/1
  gpucorr_txsim03r2_bram_data_lsb_we/1 -> mem/3(In3)
  gpucorr_txsim03r2_bram_data_lsb_data_in/1 -> mem/2(In2)
  gpucorr_txsim03r2_bram_data_lsb_addr/1 -> mem/1(In1)
  convert_we/1 -> gpucorr_txsim03r2_bram_data_lsb_we/1
  we/1 -> convert_we/1
  addr/1 -> calc_add/1(in)
  gpucorr_txsim03r2_bram_data_lsb_data_out/1 -> munge_out/1(din)
  data_in/1 -> convert_din/1
  mem/1(Out1) -> gpucorr_txsim03r2_bram_data_lsb_data_out/1

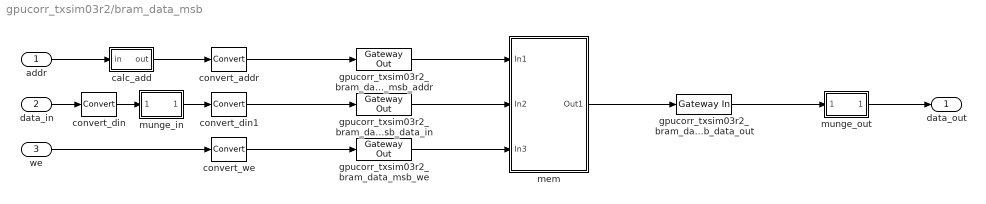
== system gpucorr_txsim03r2/bram_data_msb ==
  addr : Inport
  data_in : Inport  Port=2
  we : Inport  Port=3
  calc_add : Subsystem
  convert_addr : xbsIndex_r4/Convert  arith_type=Unsigned  n_bits=addr_width  bin_pt=0  quantization=Truncate  overflow=Wrap  latency=0  dbl_ovrd=off  pipeline=off  block_type=convert
      settings: xl_area=[0, 0, 0, 0, 0, 0, 0]
  convert_din : xbsIndex_r4/Convert  arith_type=Unsigned  n_bits=data_width  bin_pt=data_bin_pt  quantization=Truncate  overflow=Wrap  latency=0  dbl_ovrd=off  pipeline=off  block_type=convert
      settings: xl_area=[0, 0, 0, 0, 0, 0, 0]
  convert_din1 : xbsIndex_r4/Convert  arith_type=Unsigned  n_bits=data_width  bin_pt=data_bin_pt  quantization=Truncate  overflow=Wrap  latency=0  dbl_ovrd=off  pipeline=off  block_type=convert
      settings: xl_area=[0, 0, 0, 0, 0, 0, 0]
  convert_we : xbsIndex_r4/Convert  arith_type=Unsigned  n_bits=1  bin_pt=0  quantization=Truncate  overflow=Wrap  latency=0  dbl_ovrd=off  pipeline=off  block_type=convert
      settings: xl_area=[0, 0, 0, 0, 0, 0, 0]
  gpucorr_txsim03r2_bram_data_msb_addr : xbsIndex_r4/Gateway Out  hdl_port=on  timing_constraint=None  locs_specified=off  LOCs={'A5','B9','A9','C1','A3','G6','E9','A6','A7','A8','B8','B1','B3','D9','B5','B4','B6','C2'}  block_type=gatewayout
      settings: infoedit="Gateway out block.  Converts Xilinx fixed point inputs into ouputs of type Simulink integer, double, or fixed point.<P><P>Hardware notes:  In hardware these blocks become top level output ports or are discarded, depending on how they are configured."  xl_area=[0, 0, 0, 0, 0, 0, 0]  sginterface={'Nallatech'=>{'xdspkit'=>{'non_memory_mapped_port'=>'uprev_Shared_BRAM_addr'}},'Xilinx'=>{'jtaghwcosim'=>{'non_memory_mapped_port'=>'uprev_Shared_BRAM_addr'},'xdspkit'=>{'non_memory_mapped_port'=>'uprev_Shared_BRAM_addr'}}}
  gpucorr_txsim03r2_bram_data_msb_data_in : xbsIndex_r4/Gateway Out  hdl_port=on  timing_constraint=None  locs_specified=off  LOCs={'B21','B22','A22','B23','B19','C19','A20','A21','A23','B24','A24','A25','E18','D18','C18','B18'}  block_type=gatewayout
      settings: infoedit="Gateway out block.  Converts Xilinx fixed point inputs into ouputs of type Simulink integer, double, or fixed point.<P><P>Hardware notes:  In hardware these blocks become top level output ports or are discarded, depending on how they are configured."  xl_area=[0, 0, 0, 0, 0, 0, 0]  sginterface={'Nallatech'=>{'xdspkit'=>{'non_memory_mapped_port'=>'uprev_Shared_BRAM_data_in'}},'Xilinx'=>{'jtaghwcosim'=>{'non_memory_mapped_port'=>'uprev_Shared_BRAM_data_in'},'xdspkit'=>{'non_memory_mapped_port'=>'uprev_Shared_BRAM_data_in'}}}
  gpucorr_txsim03r2_bram_data_msb_data_out : xbsIndex_r4/Gateway In  arith_type=Unsigned  n_bits=data_width  bin_pt=data_bin_pt  quantization=Truncate  overflow=Wrap  period=sample_rate  dbl_ovrd=off  timing_constraint=None  locs_specified=off  LOCs={}  hdl_port=on  block_type=gatewayin
      settings: infoedit="Gateway in block.  Converts inputs of type Simulink integer, double and fixed point to  Xilinx fixed point type.<br><br>Hardware notes:  In hardware these blocks become top level input ports."  xl_area=[0, 0, 0, 0, 0, 0, 0]
  gpucorr_txsim03r2_bram_data_msb_we : xbsIndex_r4/Gateway Out  hdl_port=on  timing_constraint=None  locs_specified=off  LOCs={'A14'}  block_type=gatewayout
      settings: infoedit="Gateway out block.  Converts Xilinx fixed point inputs into ouputs of type Simulink integer, double, or fixed point.<P><P>Hardware notes:  In hardware these blocks become top level output ports or are discarded, depending on how they are configured."  xl_area=[0, 0, 0, 0, 0, 0, 0]
  mem : Subsystem
  munge_in : Subsystem  AncestorBlock=casper_library_flow_control/munge  mask(munge){divisions=1, div_size=32, order=[0]}
      mask prompts: divisions "Number of divisions"; div_size "Division size (bits)"; order "Division packing order"
      mask help: Splits an input bus into the specified number of divisions and then recombines them in the order specified (most significant division = 0,least = number divisions-1)
      mask init:
      | munge_init(gcb, ...
      |     'divisions', divisions, ...
      |     'div_size', div_size, ...
      |     'order', order);
      settings: AttributesFormatString=|
      | [0]
      | 32 bits
  munge_out : Subsystem  AncestorBlock=casper_library_flow_control/munge  mask(munge){divisions=1, div_size=32, order=[0]}
      mask prompts: divisions "Number of divisions"; div_size "Division size (bits)"; order "Division packing order"
      mask help: Splits an input bus into the specified number of divisions and then recombines them in the order specified (most significant division = 0,least = number divisions-1)
      mask init:
      | munge_init(gcb, ...
      |     'divisions', divisions, ...
      |     'div_size', div_size, ...
      |     'order', order);
      settings: AttributesFormatString=|
      | [0]
      | 32 bits
  data_out : Outport
  wires:
  convert_din/1 -> munge_in/1(din)
  convert_din1/1 -> gpucorr_txsim03r2_bram_data_msb_data_in/1
  convert_addr/1 -> gpucorr_txsim03r2_bram_data_msb_addr/1
  calc_add/1(out) -> convert_addr/1
  munge_out/1(dout) -> data_out/1
  munge_in/1(dout) -> convert_din1/1
  gpucorr_txsim03r2_bram_data_msb_we/1 -> mem/3(In3)
  gpucorr_txsim03r2_bram_data_msb_data_in/1 -> mem/2(In2)
  gpucorr_txsim03r2_bram_data_msb_addr/1 -> mem/1(In1)
  convert_we/1 -> gpucorr_txsim03r2_bram_data_msb_we/1
  we/1 -> convert_we/1
  addr/1 -> calc_add/1(in)
  gpucorr_txsim03r2_bram_data_msb_data_out/1 -> munge_out/1(din)
  data_in/1 -> convert_din/1
  mem/1(Out1) -> gpucorr_txsim03r2_bram_data_msb_data_out/1
